simulink model "mainmodel"  (R2020a)
settings: Solver=VariableStepAuto  StartTime=0.0  StopTime=10.0  RelTol=1e-3
settings Model: Creator=Bhanu  LastModifiedBy=Bhanu

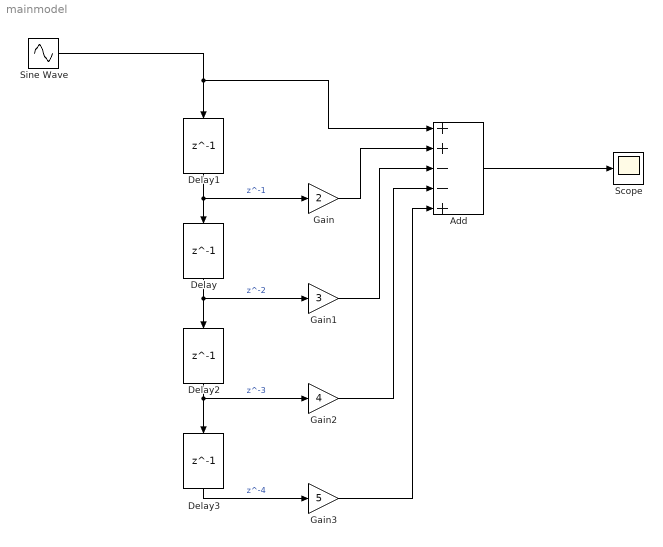
== system mainmodel ==
  Add : Sum  Inputs=++--+
  Delay{,1..3} (4 alike) : Delay  DelayLength=1  InitialCondition=0  UseCircularBuffer=on
  Gain : Gain  Gain=2
  Gain1 : Gain  Gain=3
  Gain2 : Gain  Gain=4
  Gain3 : Gain  Gain=5
  Scope : Scope
  Sine Wave : Sin  SampleTime=0
  wires:
  Delay2/1 -> Delay3/1, Gain2/1  "z^-3"
  Delay/1 -> Gain1/1, Delay2/1  "z^-2"
  Delay1/1 -> Gain/1, Delay/1  "z^-1"
  Sine Wave/1 -> Add/1, Delay1/1
  Delay3/1 -> Gain3/1  "z^-4"
  Gain/1 -> Add/2
  Gain1/1 -> Add/3
  Gain2/1 -> Add/4
  Gain3/1 -> Add/5
  Add/1 -> Scope/1
